simulink model "BajaCVTSim_SimulinkModel"  (R2025a)
settings: Solver=VariableStepAuto  StartTime=0.0  StopTime=30  RelTol=1e-2
model workspace (MAT data in the model file):
  CG = 19.90914
  Cd = 8.5
  Helix = 30
  I_high = 0.9
  I_low = 3.9
  Id_set = 1800
  LR_set = 2400
  L_link = 1.23
  RD_set = 3800
  R_gear = 6.3
  R_helix = 1.455
  R_link = 1.6
  Ramp = 18
  Rfly_max = 1.5
  Rfly_min = 1.89
  Rp_end = 2.775
  Rp_int = 0.975
  Rp_max = 0.975
  Rp_min = 2.775
  Rs_end = 2.4975
  Rs_int = 3.8025
  Rs_max = 2.4975
  Rs_min = 3.8025
  SS_set = 3000
  U = 0.13
  X_0 = 0.975
  X_max = 0.8
  Y_0 = 1.44
  Y_max = 0.8
  axle_F = 32.19442
  axle_R = 29.813464567
  eng_rpm = [1600 1800 2000 2200 2400 2600 2800 3000 3200 3400 3600 4000]
  eng_trq = [15.4 16.5 17.5 18.2 18.5 18.1 17.4 16.6 15.4 14.5 13.5 10]
  kp_lr = 43.75
  ks_lr = 21.25
  ks_tr = 0.592
  m_fly = 120
  m_link = 40
  m_ve = 600
  n_arm = 4
  phi_0 = 100
  phi_max = 40
  theta = 15
  tr = 11
libraries: fl_lib x12, sdl_lib x10, nesl_utility x10, SignalEditorBlockLib x1
settings Model: SimulationMode=accelerator  Creator=jkiss  LastModifiedBy=jkiss
settings DataIOCC: SaveFormat=Array  DSMLogging=off  ReturnWorkspaceOutputs=off

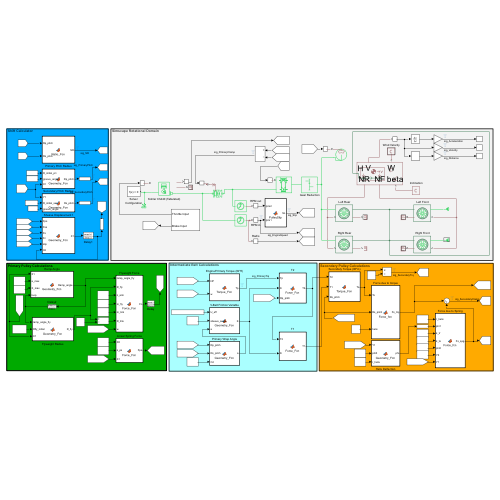
[thumbnail: Simulink's stored preview of the top-level diagram]
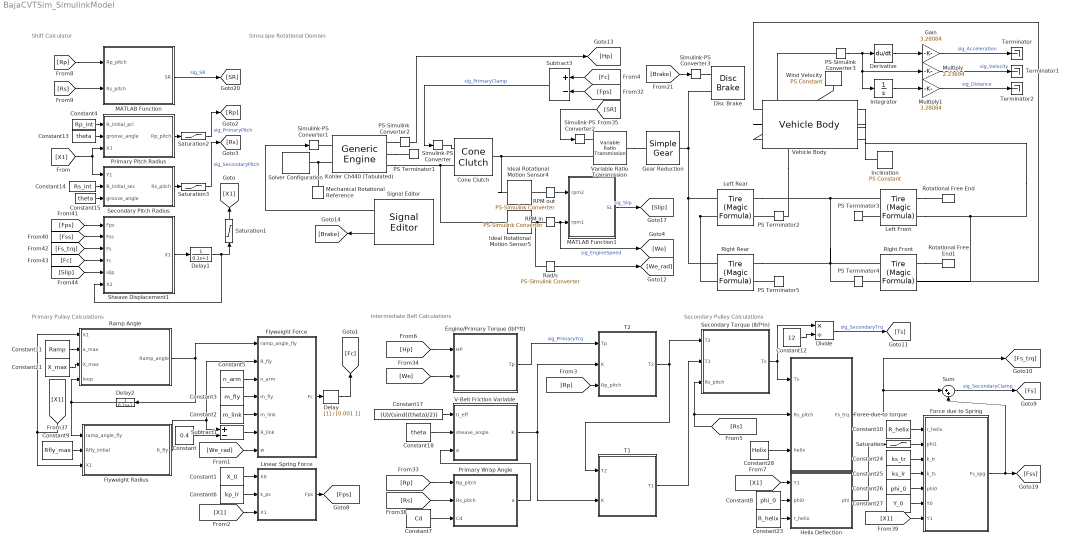
== system BajaCVTSim_SimulinkModel ==
  note: Primary Pulley Calculations
  note: Intermediate Belt Calculations
  note: Secondary Pulley Calculations
  note: Simscape Rotational Domain
  note: Shift Calculator
  Cone Clutch : sdl_lib/Clutches/Cone Clutch  d_o=Rp_end in  d_i=Rp_int in  theta=theta deg  shift_linkage=sdl.enum.shift_linkage.PS  back_stop=true  ring_hub_gap=3 mm  transl_stiffness=10e5 N/m  transl_damping=1e3 N*s/m  visc_fric_transl=100 N*s/m  direction=sdl.enum.shift_linkage_direction.positive  friction_model=sdl.enum.friction_model_TLU_thermal.fixed  mu_w_vector=[0, 100, 1000] rad/s  temperature_TLU=[280, 300, 320] K  mu_static=(U)/(sind((theta)/2))  mu_static_vector=[.4, .38, .36]  mu_coulomb=(U)/(sind((theta)/2))-0.1  mu_coulomb_vector=[.3, .22, .19]  mu_coulomb_temp_vector=[.3, .28, .25]  mu_coulomb_matrix=[.34, .32, .3; .3, .28, .25; .25, .2, .15]  mu_interp_method=simscape.enum.interpolation.linear  mu_extrap_method=simscape.enum.extrapolation.linear  w_tol=0.1 rpm  force_min=X_0*kp_lr lbf  mu_visc=0 N*m*s/rad  initial_state_locked=sdl.enum.initial_lock.unlocked  init_pos=0 mm  thermal_mass=50 kJ/K  T_init=300 K
      settings: InternalSimscapePortConfiguration="{\"Bottom\":[],\"Left\":[{\"id\":\"N\",\"label\":\"N\",\"type\":\"input\"},{\"id\":\"B\",\"label\":\"B\",\"type\":\"foundation.mechanical.rotational.rotational\"}],\"Right\":[{\"id\":\"F\",\"label\":\"F\",\"type\":\"foundation.mechanical.rotational.rotational\"}],\"Top\":[]}"
  Constant : Constant  Value=0.4
  Constant1 : Constant  Value=X_0
  Constant10 : Constant  Value=R_helix
  Constant11 : Constant  Value=Ramp
  Constant12 : Constant  Value=12
  Constant13 : Constant  Value=theta
  Constant14 : Constant  Value=Rs_int
  Constant15 : Constant  Value=theta
  Constant17 : Constant  Value=(U)/(sind((theta)/2))
  Constant18 : Constant  Value=theta
  Constant2 : Constant  Value=m_link
  Constant21 : Constant  Value=X_max
  Constant23 : Constant  Value=R_helix
  Constant24 : Constant  Value=ks_tr
  Constant25 : Constant  Value=ks_lr
  Constant26 : Constant  Value=phi_0
  Constant27 : Constant  Value=Y_0
  Constant28 : Constant  Value=Helix
  Constant3 : Constant  Value=m_fly
  Constant4 : Constant  Value=Rp_int
  Constant5 : Constant  Value=n_arm
  Constant6 : Constant  Value=kp_lr
  Constant7 : Constant  Value=Cd
  Constant8 : Constant  Value=phi_0
  Constant9 : Constant  Value=Rfly_max
  Delay : TransferFcn  Denominator=[0.001 1]
  Delay1 : TransferFcn  Denominator=[0.1 1]
  Delay2 : TransferFcn  Denominator=[0.1 1]
  Derivative : Derivative
  Disc Brake : sdl_lib/Brakes & Detents/Rotational/Disc Brake  r_mean=150 mm  bore=10 mm  n_pads=4  thermal_port=simscape.enum.thermaleffects.omit  mu_static=0.9  mu_coulomb=0.7  temperature_TLU=[280, 300, 320] K  mu_static_TLU=[.9, .8, .7]  mu_coulomb_TLU=[.8, .7, .6]  brkwy_vel=0.1 rpm  visc_coef=0 N*m*s/rad  thermal_mass=50 kJ/K  temperature_specify=off  temperature_priority=High  temperature=300 K  temperature_nominal_specify=off  temperature_nominal_value=1  temperature_nominal_unit=K
  Divide : Product  Inputs=*/
  Engine/Primary Torque (lbf*ft) : MATLAB Function  TreatAsAtomicUnit=on
  Flyweight Force : MATLAB Function  TreatAsAtomicUnit=on
  Flyweight Radius : MATLAB Function  TreatAsAtomicUnit=on
  Force due to Spring : MATLAB Function  TreatAsAtomicUnit=on
  Force due to torque : MATLAB Function  TreatAsAtomicUnit=on
  Gain : Gain  Gain=3.28084
  Gear Reduction : sdl_lib/Gears/Simple Gear  ratio=R_gear  rotation_direction=sdl.enum.shaftOutputDirection.same  friction_model=sdl.enum.gear_efficiencies_load.off  T_noload=0.1 N*m  T_nom=5 N*m  efficiency_nom=0.8  efficiency=0.8  temperature_TLU=[280, 300, 320] K  load_TLU=[1, 5, 10] N*m  efficiency_TLU=[.95, .9, .85]  efficiency_TLU2=[.85, .8, .75; .95, .9, .85; .85, .8, .7]  w_thr=0.01 rad/s  pwr_thr=0.001 W  enable_backlash=false  hardstop_model=simscape.enum.hardstop.smooth  backlash_distance=1e-3 mm  r_base=0.1 m  transition=1e-4 mm  backlash_stiffness=1e6 N/m  backlash_damping=1e3 N*s/m  coeff_rest=0.7  v_tol=0.001 m/s  f_tol=0.001 N  mu_visc=[0, 0] N*m*s/rad  thermal_mass=50 J/K  temperature_specify=off  temperature_priority=High  temperature=300 K  temperature_nominal_specify=off  temperature_nominal_value=1  temperature_nominal_unit=K  x_backlash_specify=off  x_backlash_priority=None  x_backlash=0 mm  x_backlash_nominal_specify=off  x_backlash_nominal_value=1  x_backlash_nominal_unit=mm  f_hardstop_specify=off  f_hardstop_priority=None  f_hardstop=0 N  f_hardstop_nominal_specify=off  f_hardstop_nominal_value=1  f_hardstop_nominal_unit=N  v_backlash_specify=off  v_backlash_priority=None  v_backlash=0 m/s  v_backlash_nominal_specify=off  v_backlash_nominal_value=1  v_backlash_nominal_unit=m/s
  Helix Deflection : MATLAB Function  TreatAsAtomicUnit=on
  Ideal Rotational Motion Sensor4 : fl_lib/Mechanical/Mechanical Sensors/Ideal Rotational Motion Sensor  reference=foundation.enum.MeasurementReference.absolute  acceleration_port=false  velocity_port=true  position_port=false  wrap_angle=false  offset=0 rad
      settings: InternalSimscapePortConfiguration="{\"Bottom\":[],\"Left\":[{\"id\":\"R\",\"label\":\"R\",\"type\":\"foundation.mechanical.rotational.rotational\"}],\"Right\":[{\"id\":\"W\",\"label\":\"W\",\"type\":\"output\"}],\"Top\":[]}"
  Ideal Rotational Motion Sensor5 : fl_lib/Mechanical/Mechanical Sensors/Ideal Rotational Motion Sensor  reference=foundation.enum.MeasurementReference.absolute  acceleration_port=false  velocity_port=true  position_port=false  wrap_angle=false  offset=0 rad
      settings: InternalSimscapePortConfiguration="{\"Bottom\":[],\"Left\":[{\"id\":\"R\",\"label\":\"R\",\"type\":\"foundation.mechanical.rotational.rotational\"}],\"Right\":[{\"id\":\"W\",\"label\":\"W\",\"type\":\"output\"}],\"Top\":[]}"
  Inclination : fl_lib/Physical Signals/Sources/PS Constant  constant=0 rad
  Integrator : Integrator
  Kohler Ch440 (Tabulated) : sdl_lib/Engines & Motors/Generic Engine  input_type=sdl.enum.GenericEngineInputType.NormalizedThrottle  model_parameterization=sdl.enum.engineParameterization.torque  engine_type=sdl.enum.engineType.SI  Trq_max=380 N*m  w_Trq_max=4300 rpm  P_max=9.48 HP_DIN  w_P_max=3000 rpm  w_max=3900 rpm  w_min=0 rpm  w_tab=eng_rpm rpm  trq_tab=eng_trq ft*lb  pwr_tab=[3, 3.2, 3.5, 3.7, 4, 4.7, 5.8, 6.8, 7.6, 8.5, 9, 9.3, 9.5, 9.45, 9.4, 9.3 7] HP_DIN  interp_method=simscape.enum.interpolation.smooth  w_thr=500 rpm  model_inertia=sdl.enum.model_inertia.on  inertia=0.001 kg*m^2  initial_velocity=Id_set rpm  model_time_constant=sdl.enum.lagOffOn.off  time_constant=1 s  initial_normalized_throttle=0  fc_model=sdl.enum.fuel_consumption_model.FuelOff  fc_per_rev=25 mg/rev  fc_w_tab=[1000, 2000, 3000, 4000, 5000, 6000] rpm  fc_trq_tab=[0, 80, 160, 200, 240, 320, 360, 400] N*m  fc_tab=[.5, .9, 1.4, 1.6, 1.9, 2.7, 3.4, 4.4; 1, 1.7, 2.7, 3.1, 3.6, 5, 6, 7.4; 1.4, 2.7, 4, 4.8, 5.6, 7.5, 8.5, 10.5; 2, 3.6, 5.8, 6.7, 8, 10.4, 11.7, 13.3; 2.5, 4.8, 7.9, 9.4, 10.8, 14, 16.2, 18.6; 3.1, 6, 10.3, 11.9, 13.8, 18.4, 22, 26.5] g/s  bmep_tab=[0, 250, 500, 625, 750, 1000, 1150, 1250] kPa  bsfc_tab=[410, 380, 300, 280, 270, 290, 320, 380; 410, 370, 290, 270, 260, 270, 285, 320; 415, 380, 290, 275, 265, 270, 270, 300; 420, 390, 310, 290, 285, 280, 280, 285; 430, 410, 340, 320, 310, 300, 310, 320; 450, 430, 370, 340, 330, 330, 350, 380] g/(hr*kW)  fc_interp_method=simscape.enum.interpolation.linear  displaced_volume=400 cm^3  rev_per_cycle=2  idle_speed=true  idle_speed_reference=Id_set rpm  tau_controller=1 s  idle_w_thr=1 rpm  redline=true  redline_speed=RD_set + 200 rpm  tau_redline=0.01 s  redline_w_thr=10 rpm
      settings: InternalSimscapePortConfiguration="{\"Bottom\":[],\"Left\":[{\"id\":\"ThrNorm\",\"label\":\"Thr\",\"type\":\"input\"},{\"id\":\"B\",\"label\":\"B\",\"type\":\"foundation.mechanical.rotational.rotational\"}],\"Right\":[{\"id\":\"P\",\"label\":\"P\",\"type\":\"output\"},{\"id\":\"FC\",\"label\":\"FC\",\"type\":\"output\"},{\"id\":\"F\",\"label\":\"F\",\"type\":\"foundation.mechanical.rotational.rotational\"}],\"Top\":[]}"
  Left Front : sdl_lib/Tires & Vehicles/Tire (Magic Formula)  parameterization=1  F_z1=2060 N  F_x1=1260 N  kappa1=1  B_m=10  C_m=1.9  D_m=1  E_m=0.97  fz0=2060 N  p_Cx=1.685  p_Dx=[1.21, -.037]  p_Ex=[.344, .095, -.02, 0]  p_Kx=[21.51, -.163, .245]  p_Hx=[-.002, .002]  p_Vx=[0, 0]  rolling_radius_model=sdl.enum.RollingRadiusParameterization.Constant  r_e=tr in  r_0=0.3 m  breff=8.39  dreff=0.26  freff=0.074  q_re0=0.99  q_v1=0.008  longvl=17 m/s  cz=5e5 N/m  model_resistance=false  resistance_model=1  coeff=0.001  p_tire=250e3 Pa  alpha=-0.003  beta=0.97  coeff_a=84e-4  coeff_b=6.2e-4 s/m  coeff_c=1.6e-4 s^2/m^2  p_tire0=240e3 Pa  fz0_resistance=4000 N  vH0=16 m/s  q_Sy=[.0082, 0, .0014, .001, 0, 0, 1.08, -.5]  v_thr=0.1 m/s  enable_scaling_coefficients=false  lfzO=1  lcx=1  lmux=1  lex=1  lkx=1  lhx=1  lvx=1  lmy=1  model_compliance=0  stiffness=1e6 N/m  damping=1000 N/(m/s)  model_inertia=sdl.enum.model_inertia.off  inertia=1e-2 kg*m^2  initial_velocity=0 rpm  vxlow=0.1 m/s  v_tr_thr=0.1*(0.1) m/s  kpumin=-5  kpumax=5
  Left Rear : sdl_lib/Tires & Vehicles/Tire (Magic Formula)  parameterization=sdl.enum.magic_tire_model.peak  F_z1=2060 N  F_x1=1260 N  kappa1=1  B_m=10  C_m=1.9  D_m=1  E_m=0.97  fz0=4000 N  p_Cx=1.685  p_Dx=[1.21, -.037]  p_Ex=[.344, .095, -.02, 0]  p_Kx=[21.51, -.163, .245]  p_Hx=[-.002, .002]  p_Vx=[0, 0]  rolling_radius_model=sdl.enum.RollingRadiusParameterization.Constant  r_e=tr in  r_0=0.3 m  breff=8.39  dreff=0.26  freff=0.074  q_re0=0.99  q_v1=0.008  longvl=17 m/s  cz=5e5 N/m  model_resistance=false  resistance_model=1  coeff=0.001  p_tire=250e3 Pa  alpha=-0.003  beta=0.97  coeff_a=84e-4  coeff_b=6.2e-4 s/m  coeff_c=1.6e-4 s^2/m^2  p_tire0=240e3 Pa  fz0_resistance=4000 N  vH0=16 m/s  q_Sy=[.0082, 0, .0014, .001, 0, 0, 1.08, -.5]  v_thr=0.1 m/s  enable_scaling_coefficients=false  lfzO=1  lcx=1  lmux=1  lex=1  lkx=1  lhx=1  lvx=1  lmy=1  model_compliance=0  stiffness=1e6 N/m  damping=1000 N/(m/s)  model_inertia=sdl.enum.model_inertia.off  inertia=1e-2 kg*m^2  initial_velocity=0 rpm  vxlow=0.1 m/s  v_tr_thr=0.1 m/s  kpumin=-5  kpumax=5
  Linear Spring Force : MATLAB Function  TreatAsAtomicUnit=on
  MATLAB Function : MATLAB Function  TreatAsAtomicUnit=on
  MATLAB Function1 : MATLAB Function  TreatAsAtomicUnit=on
  Mechanical Rotational Reference : fl_lib/Mechanical/Rotational Elements/Mechanical Rotational Reference
  Multiply : Gain  Gain=2.23694
  Multiply1 : Gain  Gain=3.28084
  PS Terminator{1..5} (5 alike) : fl_lib/Physical Signals/Sinks/PS Terminator
  PS-Simulink Converter2 : nesl_utility/PS-Simulink Converter  PhysicalDomain=network_engine_domain  SubClassName=ps_output  LeftPortType=input  RightPortType=output  PseudoPeriodic=off  Frequencies=[]  VectorFormat=inherit  Unit=HP_DIN  AffineConversion=off
  PS-Simulink Converter3 : nesl_utility/PS-Simulink Converter  PhysicalDomain=network_engine_domain  SubClassName=ps_output  LeftPortType=input  RightPortType=output  PseudoPeriodic=off  Frequencies=[]  VectorFormat=1-D array  Unit=m/s  AffineConversion=off
  Primary Pitch Radius : MATLAB Function  TreatAsAtomicUnit=on
  Primary Wrap Angle : MATLAB Function  TreatAsAtomicUnit=on
  RPM in : nesl_utility/PS-Simulink Converter  PhysicalDomain=network_engine_domain  SubClassName=ps_output  LeftPortType=input  RightPortType=output  PseudoPeriodic=off  Frequencies=[]  VectorFormat=inherit  Unit=rpm  AffineConversion=off
  RPM out : nesl_utility/PS-Simulink Converter  PhysicalDomain=network_engine_domain  SubClassName=ps_output  LeftPortType=input  RightPortType=output  PseudoPeriodic=off  Frequencies=[]  VectorFormat=inherit  Unit=rpm  AffineConversion=off
  Rad/s : nesl_utility/PS-Simulink Converter  PhysicalDomain=network_engine_domain  SubClassName=ps_output  LeftPortType=input  RightPortType=output  PseudoPeriodic=off  Frequencies=[]  VectorFormat=inherit  Unit=rad/s  AffineConversion=off
  Ramp Angle : MATLAB Function  TreatAsAtomicUnit=on
  Right Front : sdl_lib/Tires & Vehicles/Tire (Magic Formula)  parameterization=1  F_z1=2060 N  F_x1=1260 N  kappa1=1  B_m=10  C_m=1.9  D_m=1  E_m=0.97  fz0=4000 N  p_Cx=1.685  p_Dx=[1.21, -.037]  p_Ex=[.344, .095, -.02, 0]  p_Kx=[21.51, -.163, .245]  p_Hx=[-.002, .002]  p_Vx=[0, 0]  rolling_radius_model=sdl.enum.RollingRadiusParameterization.Constant  r_e=tr in  r_0=0.3 m  breff=8.39  dreff=0.26  freff=0.074  q_re0=0.99  q_v1=0.008  longvl=17 m/s  cz=5e5 N/m  model_resistance=false  resistance_model=1  coeff=0.001  p_tire=250e3 Pa  alpha=-0.003  beta=0.97  coeff_a=84e-4  coeff_b=6.2e-4 s/m  coeff_c=1.6e-4 s^2/m^2  p_tire0=240e3 Pa  fz0_resistance=4000 N  vH0=16 m/s  q_Sy=[.0082, 0, .0014, .001, 0, 0, 1.08, -.5]  v_thr=0.1 m/s  enable_scaling_coefficients=false  lfzO=1  lcx=1  lmux=1  lex=1  lkx=1  lhx=1  lvx=1  lmy=1  model_compliance=0  stiffness=1e6 N/m  damping=1000 N/(m/s)  model_inertia=sdl.enum.model_inertia.off  inertia=1e-2 kg*m^2  initial_velocity=0 rpm  vxlow=0.1 m/s  v_tr_thr=0.1*(0.1) m/s  kpumin=-5  kpumax=5
  Right Rear : sdl_lib/Tires & Vehicles/Tire (Magic Formula)  parameterization=sdl.enum.magic_tire_model.peak  F_z1=2060 N  F_x1=1260 N  kappa1=1  B_m=10  C_m=1.9  D_m=1  E_m=0.97  fz0=4000 N  p_Cx=1.685  p_Dx=[1.21, -.037]  p_Ex=[.344, .095, -.02, 0]  p_Kx=[21.51, -.163, .245]  p_Hx=[-.002, .002]  p_Vx=[0, 0]  rolling_radius_model=sdl.enum.RollingRadiusParameterization.Constant  r_e=tr in  r_0=0.3 m  breff=8.39  dreff=0.26  freff=0.074  q_re0=0.99  q_v1=0.008  longvl=17 m/s  cz=5e5 N/m  model_resistance=false  resistance_model=1  coeff=0.001  p_tire=250e3 Pa  alpha=-0.003  beta=0.97  coeff_a=84e-4  coeff_b=6.2e-4 s/m  coeff_c=1.6e-4 s^2/m^2  p_tire0=240e3 Pa  fz0_resistance=4000 N  vH0=16 m/s  q_Sy=[.0082, 0, .0014, .001, 0, 0, 1.08, -.5]  v_thr=0.1 m/s  enable_scaling_coefficients=false  lfzO=1  lcx=1  lmux=1  lex=1  lkx=1  lhx=1  lvx=1  lmy=1  model_compliance=0  stiffness=1e6 N/m  damping=1000 N/(m/s)  model_inertia=sdl.enum.model_inertia.off  inertia=1e-2 kg*m^2  initial_velocity=0 rpm  vxlow=0.1 m/s  v_tr_thr=0.1 m/s  kpumin=-5  kpumax=5
  Rotational Free End : fl_lib/Mechanical/Rotational Elements/Rotational Free End  w_specify=off  w_priority=None  w=0 rad/s  w_nominal_specify=off  w_nominal_value=1  w_nominal_unit=rad/s
  Rotational Free End1 : fl_lib/Mechanical/Rotational Elements/Rotational Free End  w_specify=off  w_priority=None  w=0 rad/s  w_nominal_specify=off  w_nominal_value=1  w_nominal_unit=rad/s
  Saturation : Saturate  UpperLimit=phi_0 + phi_max  LowerLimit=phi_0
  Saturation1 : Saturate  UpperLimit=X_max  LowerLimit=0
  Saturation2 : Saturate  UpperLimit=Rp_end  LowerLimit=Rp_int
  Saturation3 : Saturate  UpperLimit=Rs_int  LowerLimit=Rs_end
  Secondary Pitch Radius : MATLAB Function  TreatAsAtomicUnit=on
  Secondary Torque (lbf*in) : MATLAB Function  TreatAsAtomicUnit=on
  Sheave Displacement1 : MATLAB Function  TreatAsAtomicUnit=on
  Signal Editor : SignalEditorBlockLib/Signal Editor  FileName=BajaCVTSim_ThrottleInputs.mat  ActiveScenario=IDLE_50  ActiveSignal=Throttle Input  IsBus=off  OutputBusObjectStr=Bus: BusObject  SampleTime=0  ZeroCross=off  OutputAfterFinalValue=Holding final value  Unit=inherit  PreserveSignalName=on  ApplySigPropsToAllScenarios=on  ApplySigPropsToAllSignals=off  SignalPropertySource=Dialog parameters
  Simulink-PS Converter : nesl_utility/Simulink-PS Converter  PhysicalDomain=network_engine_domain  SubClassName=ps_input  LeftPortType=input  RightPortType=output  PseudoPeriodic=off  Frequencies=[]  NoiseDistribution=none  NoiseParameters=[]  Unit=lbf  AffineConversion=off  FilteringAndDerivatives=provide  SimscapeFilterOrder=1  InputFilterTimeConstant=0.001  UdotUserProvided=0
  Simulink-PS Converter1 : nesl_utility/Simulink-PS Converter  PhysicalDomain=network_engine_domain  SubClassName=ps_input  LeftPortType=input  RightPortType=output  PseudoPeriodic=off  Frequencies=[]  NoiseDistribution=none  NoiseParameters=[]  Unit=1  AffineConversion=off  FilteringAndDerivatives=provide  SimscapeFilterOrder=1  InputFilterTimeConstant=0.001  UdotUserProvided=0
  Simulink-PS Converter2 : nesl_utility/Simulink-PS Converter  PhysicalDomain=network_engine_domain  SubClassName=ps_input  LeftPortType=input  RightPortType=output  PseudoPeriodic=off  Frequencies=[]  NoiseDistribution=none  NoiseParameters=[]  Unit=1  AffineConversion=off  FilteringAndDerivatives=provide  SimscapeFilterOrder=1  InputFilterTimeConstant=0.001  UdotUserProvided=0
  Simulink-PS Converter3 : nesl_utility/Simulink-PS Converter  PhysicalDomain=network_engine_domain  SubClassName=ps_input  LeftPortType=input  RightPortType=output  PseudoPeriodic=off  Frequencies=[]  NoiseDistribution=none  NoiseParameters=[]  Unit=1  AffineConversion=off  FilteringAndDerivatives=provide  SimscapeFilterOrder=1  InputFilterTimeConstant=0.001  UdotUserProvided=0
  Solver Configuration : nesl_utility/Solver Configuration  PhysicalDomain=network_engine_domain  SubClassName=solver  LeftPortType=input  RightPortType=generic  Tones=[]  Harmonics=[]  SimulateNoise=off  Profile=off  UseLocalSampling=off  EnableSwitchedLinearOptims=on  FrequencyDomain=off  UseCCode=off  RelTol=0.001  AbsTol=1e-06  MinStep=1e-09  ToWorkspace=off  RevertToSquareIcSolve=off  NumHomotopyIterations=100  PhasorMode=off  PhasorModeNumHarmonics=1  ConsistencySolver=NEWTON_XTOL_AFTER_FTOL  IndexReductionMethod=DerivativeReplacement  DoDC=off  ResidualTolerance=1e-09  ConsistencyTolSource=GLOBAL  ConsistencyAbsTol=0.001  ConsistencyRelTol=0.001  ConsistencyTolFactor=0.001  UseLocalSolver=off  LocalSolverChoice=NE_BACKWARD_EULER_ADVANCER  ResolveIndetEquations=on  FunctionEvalNumThread=1  LocalSolverSampleTime=0.001  DoFixedCost=off  MaxNonlinIter=3  MaxModeIter=2  ComputeImpulses=off  ImpulseIterations=2  LinearAlgebra=auto  LinearAlgebraNumThread=0  EquationFormulation=NE_TIME_EF  DelaysMemoryBudget=1024  AutomaticFiltering=on  FilteringTimeConstant=0.001  PartitionStorageMethod=AS_NEEDED  PartitionMemoryBudget=1024  PartitionMethod=ROBUST  MultibodyUseLocalSolver=off  MultibodyLocalSolverChoice=ODE1  MultibodyLocalSolverSampleTime=0.001
  Subtract1 : Sum  Inputs=+-
  Subtract3 : Sum  Inputs=+-
  Sum : Sum  Inputs=|++
  T1 : MATLAB Function  TreatAsAtomicUnit=on
  T2 : MATLAB Function  TreatAsAtomicUnit=on
  Terminator : Terminator
  Terminator1 : Terminator
  Terminator2 : Terminator
  V-Belt Friction Variable : MATLAB Function  TreatAsAtomicUnit=on
  Variable Ratio Transmission : sdl_lib/Couplings & Drives/Variable Ratio Transmission  rotation_direction=sdl.enum.shaftOutputDirection.same  kp=1e3 N*m/rad  kv=10 N*m*s/rad  initial_torque=0 N*m  ratio_thr=0.01  losses_model=sdl.enum.lossesOffOn.off  efficiency=0.8  pwr_thr=0.001 W  mu_visc=[0, 0] N*m*s/rad
      settings: InternalSimscapePortConfiguration="{\"Bottom\":[],\"Left\":[{\"id\":\"ratio\",\"label\":\"r\",\"type\":\"input\"},{\"id\":\"B\",\"label\":\"B\",\"type\":\"foundation.mechanical.rotational.rotational\"}],\"Right\":[{\"id\":\"F\",\"label\":\"F\",\"type\":\"foundation.mechanical.rotational.rotational\"}],\"Top\":[]}"
  Vehicle Body : sdl_lib/Tires & Vehicles/Vehicle Body  mass=m_ve lbm  n_w=2  x_f=axle_F in  x_r=axle_R in  y_c=CG+10 in  mass_var=simscape.enum.onoff.off  g=32.2 ft/s^2  liftoff_warning=0  area=.735482 m^2  Cd_var=false  Cd=1.92  rho=1.18 kg/m^3  model_pitch=0  inertia=4000 kg*m^2  suspension_model=1  k_f=1e4 N/m  b_f=1e4 N/(m/s)  k_r=1e4 N/m  b_r=1e4 N/(m/s)  k_f_TLU=[-2000, -1000, 0, 1000, 2000] N  x_f_TLU=[-.4, -.2, 0, .2, .4] m  b_f_TLU=[-200, -100, 0, 100, 200] N  v_f_TLU=[-4, -2, 0, 2, 4] m/s  k_r_TLU=[-2000, -1000, 0, 1000, 2000] N  x_r_TLU=[-.4, -.2, 0, .2, .4] m  b_r_TLU=[-200, -100, 0, 100, 200] N  v_r_TLU=[-4, -2, 0, 2, 4] m/s  interp_method=simscape.enum.interpolation.linear  extrap_method=simscape.enum.extrapolation.linear  model_hardstop=0  upper_bound_f=.25 m  lower_bound_f=-.25 m  stop_k_f=1e6 N/m  stop_b_f=150 N/(m/s)  upper_bound_r=.25 m  lower_bound_r=-.25 m  stop_k_r=1e6 N/m  stop_b_r=150 N/(m/s)  initial_pitch=0 rad  initial_pitch_rate=0 rad/s  v_specify=on  v_priority=High  v=0 m/s  v_nominal_specify=off  v_nominal_value=1  v_nominal_unit=m/s
      settings: InternalSimscapePortConfiguration="{\"Bottom\":[{\"id\":\"NR\",\"label\":\"NR\",\"type\":\"output\"},{\"id\":\"NF\",\"label\":\"NF\",\"type\":\"output\"},{\"id\":\"beta\",\"label\":\"beta\",\"type\":\"input\"}],\"Left\":[{\"id\":\"H\",\"label\":\"H\",\"type\":\"foundation.mechanical.translational.translational\"}],\"Right\":[],\"Top\":[{\"id\":\"V\",\"label\":\"V\",\"type\":\"output\"},{\"id\":\"wind\",\"label\":\"W\",\"type\":\"input\"}]}"
  Wind Velocity : fl_lib/Physical Signals/Sources/PS Constant  constant=0
  wires:
  Signal Editor/2 -> [Brake]
  [Fc] -> Subtract3/1
  MATLAB Function1/1(SL) -> [Slip]  "sig_Slip"
  RPM out/1 -> MATLAB Function1/1(rpm2)
  RPM in/1 -> [We], MATLAB Function1/2(rpm1)  "sig_EngineSpeed"
  Constant5/1 -> Flyweight Force/3(n_arm)
  Constant3/1 -> Flyweight Force/4(m_fly)
  Constant2/1 -> Flyweight Force/5(m_link)
  Flyweight Radius/1(R_fly) -> Subtract1/1, Flyweight Force/2(R_fly)
  Subtract1/1 -> Flyweight Force/6(R_link)
  Constant/1 -> Subtract1/2
  Constant9/1 -> Flyweight Radius/2(Rfly_initial)
  [X1] -> Ramp Angle/1(X1), Flyweight Radius/3(X1)
  Ramp Angle/1(Ramp_angle) -> Flyweight Force/1(ramp_angle_fly), Delay2/1
  Constant11/1 -> Ramp Angle/2(a_max)
  Constant21/1 -> Ramp Angle/3(X_max)
  [X1] -> Linear Spring Force/3(X1)
  Constant1/1 -> Linear Spring Force/1(X0)
  Constant6/1 -> Linear Spring Force/2(k_ps)
  Flyweight Force/1(Fc) -> Delay/1
  Rad/s/1 -> [We_rad]
  T2/1(T2) -> T1/1(T2), Secondary Torque (lbf*in)/1(T2)
  Delay/1 -> [Fc]
  T1/1(T1) -> Secondary Torque (lbf*in)/2(T1)
  Linear Spring Force/1(Fps) -> [Fps]
  [Rs] -> Primary Wrap Angle/2(Rs_pitch)
  [Rp] -> Primary Wrap Angle/1(Rp_pitch)
  [Rs] -> Secondary Torque (lbf*in)/3(Rs_pitch), Force due to torque/2(Rs_pitch)
  [Rp] -> T2/3(Rp_pitch)
  Constant10/1 -> Force due to Spring/1(r_helix)
  Constant8/1 -> Helix Deflection/2(phi0)
  Constant23/1 -> Helix Deflection/3(r_helix)
  Helix Deflection/1(phi) -> Saturation/1
  Constant18/1 -> V-Belt Friction Variable/2(sheave_angle)
  Constant26/1 -> Force due to Spring/5(phi0)
  Constant24/1 -> Force due to Spring/3(k_tr)
  Constant25/1 -> Force due to Spring/4(k_ts)
  Constant27/1 -> Force due to Spring/6(Y0)
  Constant7/1 -> Primary Wrap Angle/3(Cd)
  Signal Editor/1 -> Simulink-PS Converter1/1
  [Fps] -> Subtract3/2
  Subtract3/1 -> Simulink-PS Converter/1  "sig_PrimaryClamp"
  [We] -> Engine/Primary Torque (lbf*ft)/2(w)
  PS-Simulink Converter2/1 -> [Hp]
  [Hp] -> Engine/Primary Torque (lbf*ft)/1(HP)
  [SR] -> Simulink-PS Converter2/1
  PS-Simulink Converter3/1 -> Derivative/1, Integrator/1, Multiply/1
  Multiply/1 -> Terminator1/1  "sig_Velocity"
  Integrator/1 -> Multiply1/1
  Multiply1/1 -> Terminator2/1  "sig_Distance"
  [Brake] -> Simulink-PS Converter3/1
  [We_rad] -> Flyweight Force/7(w)
  Primary Wrap Angle/1(a) -> V-Belt Friction Variable/3(a)
  Constant17/1 -> V-Belt Friction Variable/1(U_eff)
  V-Belt Friction Variable/1(K) -> T1/2(K), T2/2(K)
  Engine/Primary Torque (lbf*ft)/1(Tp) -> T2/1(Tp)  "sig_PrimaryTrq"
  Divide/1 -> [Ts]  "sig_SecondaryTrq"
  [X1] -> Helix Deflection/1(Y1)
  Saturation/1 -> Force due to Spring/2(phi1)
  Force due to torque/1(Fs_trq) -> [Fs_trq], Sum/1
  Sum/1 -> [Fs]  "sig_SecondaryClamp"
  Force due to Spring/1(Fs_spg) -> [Fss], Sum/2
  [X1] -> Force due to Spring/7(Y1)
  [Fss] -> Sheave Displacement1/2(Fss)
  [Fs_trq] -> Sheave Displacement1/3(Fs)
  [Fps] -> Sheave Displacement1/1(Fps)
  [Fc] -> Sheave Displacement1/4(Fc)
  [Slip] -> Sheave Displacement1/5(slip)
  Delay1/1 -> Sheave Displacement1/6(X2), Saturation1/1
  Sheave Displacement1/1(X1) -> Delay1/1
  Constant13/1 -> Primary Pitch Radius/2(groove_angle)
  Primary Pitch Radius/1(Rp_pitch) -> Saturation2/1
  Constant4/1 -> Primary Pitch Radius/1(R_initial_pri)
  Constant14/1 -> Secondary Pitch Radius/2(R_initial_sec)
  Constant15/1 -> Secondary Pitch Radius/3(groove_angle)
  Secondary Pitch Radius/1(Rs_pitch) -> Saturation3/1
  MATLAB Function/1(SR) -> [SR]  "sig_SR"
  Constant28/1 -> Force due to torque/3(helix)
  Delay2/1 -> Ramp Angle/4(loop), Flyweight Radius/1(ramp_angle_fly)
  Secondary Torque (lbf*in)/1(Ts) -> Divide/1, Force due to torque/1(Ts)
  Constant12/1 -> Divide/2
  Derivative/1 -> Gain/1
  Gain/1 -> Terminator/1  "sig_Acceleration"
  Saturation2/1 -> [Rp]  "sig_PrimaryPitch"
  Saturation3/1 -> [Rs]  "sig_SecondaryPitch"
  [X1] -> Primary Pitch Radius/3(X1), Secondary Pitch Radius/1(Y1)
  [Rs] -> MATLAB Function/2(Rs_pitch)
  [Rp] -> MATLAB Function/1(Rp_pitch)
  Saturation1/1 -> [X1]
  connections:
  Kohler Ch440 (Tabulated)/LConn2 -- Solver Configuration/RConn1 -- Mechanical Rotational Reference/LConn1
  Ideal Rotational Motion Sensor5/LConn1 -- Kohler Ch440 (Tabulated)/RConn3 -- Cone Clutch/LConn2
  Rad/s/LConn1 -- Ideal Rotational Motion Sensor5/RConn1 -- RPM in/LConn1
  Ideal Rotational Motion Sensor4/LConn1 -- Cone Clutch/RConn1 -- Variable Ratio Transmission/LConn2
  Simulink-PS Converter/RConn1 -- Cone Clutch/LConn1
  RPM out/LConn1 -- Ideal Rotational Motion Sensor4/RConn1
  Right Rear/LConn2 -- Left Rear/LConn2 -- Gear Reduction/RConn1 -- Disc Brake/LConn2
  Simulink-PS Converter2/RConn1 -- Variable Ratio Transmission/LConn1
  Variable Ratio Transmission/RConn1 -- Gear Reduction/LConn1
  Kohler Ch440 (Tabulated)/LConn1 -- Simulink-PS Converter1/RConn1
  Kohler Ch440 (Tabulated)/RConn1 -- PS-Simulink Converter2/LConn1
  Kohler Ch440 (Tabulated)/RConn2 -- PS Terminator1/LConn1
  Left Rear/LConn1 -- Vehicle Body/RConn1 -- Right Rear/LConn1
  Right Front/RConn2 -- Vehicle Body/LConn1 -- Right Rear/RConn2 -- Left Rear/RConn2 -- Left Front/RConn2
  Left Front/LConn1 -- Vehicle Body/RConn2 -- Right Front/LConn1
  Vehicle Body/RConn3 -- Inclination/RConn1
  Left Front/RConn1 -- PS Terminator3/LConn1
  Simulink-PS Converter3/RConn1 -- Disc Brake/LConn1
  Left Front/LConn2 -- Rotational Free End/LConn1
  Right Front/RConn1 -- PS Terminator4/LConn1
  Vehicle Body/LConn3 -- Wind Velocity/RConn1
  Right Front/LConn2 -- Rotational Free End1/LConn1
  Vehicle Body/LConn2 -- PS-Simulink Converter3/LConn1
  PS Terminator2/LConn1 -- Left Rear/RConn1
  PS Terminator5/LConn1 -- Right Rear/RConn1

== matlab function BajaCVTSim_SimulinkModel/Linear Spring Force ==
  data: X0 input; k_ps input; X1 input; Fps output
function Fps = Force_Fcn(X0,k_ps,X1)

Fps = k_ps*(X0 + X1);

end

== matlab function BajaCVTSim_SimulinkModel/Secondary Torque (lbf*in) ==
  data: T2 input; Ts output; T1 input; Rs_pitch input
function Ts = Torque_Fcn(T2,T1,Rs_pitch)

Ts = (T1-T2)*Rs_pitch; %lbf*in

end

== matlab function BajaCVTSim_SimulinkModel/Force due to torque ==
  data: Ts input; Rs_pitch input; helix input; Fs_trq output
function Fs_trq = Force_fcn(Ts,Rs_pitch,helix)

Fs_trq = (Ts/Rs_pitch)*tand(helix);

end

== matlab function BajaCVTSim_SimulinkModel/Force due to Spring ==
  data: r_helix input; phi1 input; k_tr input; k_ts input; Fs_spg output; phi0 input; Y0 input; Y1 input
function Fs_spg = Force_fcn(r_helix,phi1,k_tr,k_ts,phi0,Y0,Y1)

Fs_spg = (k_tr*(phi0 + phi1))/(2*r_helix) + (k_ts*(Y0 + Y1));

end

== matlab function BajaCVTSim_SimulinkModel/Flyweight Force ==
  data: ramp_angle_fly input; R_fly input; n_arm input; m_fly input; m_link input; R_link input; w input; Fc output
function Fc = Force_Fcn(ramp_angle_fly,R_fly,n_arm,m_fly,m_link,R_link,w)

Fc = (((m_fly/14593.89567)*n_arm*(R_fly/12) + (m_link/14593.89567)*n_arm*(R_link/12))*(w^2))*tand(ramp_angle_fly);

end

== matlab function BajaCVTSim_SimulinkModel/Sheave Displacement1 ==
  data: Fps input; Fss input; Fs input; Fc input; slip input; X1 output; X2 input
function X1 = Geometry_Fcn(Fps,Fss,Fs,Fc,slip,X2)
    if slip <= 5
        if X2 >= 0.2
            if Fc-Fps > Fs + Fss
                X1 = X2 + 0.0799;
            else
                X1 = X2;
            end
        elseif X2 >= 0.35
            if Fc-Fps > Fs + Fss
                X1 = X2 + 0.01;
            else
                X1 = X2;
            end
        else
            if Fc-Fps > Fs + Fss
                X1 = X2 + 0.08;
            else
                X1 = X2;
            end
        end
    else
        X1 = 0;
    end
end

== matlab function BajaCVTSim_SimulinkModel/Primary Pitch Radius ==
  data: R_initial_pri input; groove_angle input; X1 input; Rp_pitch output
function Rp_pitch = Geometry_Fcn(R_initial_pri,groove_angle,X1)

Rp_pitch = R_initial_pri + (X1)/tand(groove_angle);

end

== matlab function BajaCVTSim_SimulinkModel/Secondary Pitch Radius ==
  data: Y1 input; R_initial_sec input; Rs_pitch output; groove_angle input
function Rs_pitch = Geometry_Fcn(Y1,R_initial_sec,groove_angle)

Rs_pitch = R_initial_sec - (Y1)/tand(groove_angle);

end

== matlab function BajaCVTSim_SimulinkModel/MATLAB Function ==
  data: Rp_pitch input; SR output; Rs_pitch input
function SR = Ratio_Fcn(Rp_pitch,Rs_pitch)

SR = Rs_pitch/Rp_pitch;

end

== matlab function BajaCVTSim_SimulinkModel/Helix Deflection ==
  data: Y1 input; phi0 input; r_helix input; phi output
function phi = Geometry_Fcn(Y1,phi0,r_helix)

phi = 2*(90 - acosd(Y1/r_helix)) + phi0;

end

== matlab function BajaCVTSim_SimulinkModel/Primary Wrap Angle ==
  data: Rp_pitch input; a output; Rs_pitch input; Cd input
function a = Geometry_Fcn(Rp_pitch,Rs_pitch,Cd)

a = pi + 2*asin((Rs_pitch-Rp_pitch)/Cd);

end

== matlab function BajaCVTSim_SimulinkModel/V-Belt Friction Variable ==
  data: U_eff input; sheave_angle input; a input; K output
function K = Geometry_Fcn(U_eff,sheave_angle,a)

K = exp((U_eff*a)/sind(sheave_angle));

end

== matlab function BajaCVTSim_SimulinkModel/T1 ==
  data: T2 input; T1 output; K input
function T1 = Force_Fcn(T2,K)

T1 = T2*K;

end

== matlab function BajaCVTSim_SimulinkModel/MATLAB Function1 ==
  data: rpm2 input; rpm1 input; SL output
function SL = PulleySlip(rpm2,rpm1)

SL = ((rpm1-rpm2)/rpm1) * 100;

end

== matlab function BajaCVTSim_SimulinkModel/T2 ==
  data: Tp input; T2 output; K input; Rp_pitch input
function T2 = Force_Fcn(Tp,K,Rp_pitch)

T2 = (Tp*12)/(Rp_pitch*(K-1));

end

== matlab function BajaCVTSim_SimulinkModel/Ramp Angle ==
  data: X1 input; a_max input; X_max input; Ramp_angle output; loop input
function Ramp_angle = Geometry_Fcn(X1,a_max,X_max,loop)
if X1 >= X_max*0.25
    Ramp_angle = a_max - exp(-4*(0.2-X1)) + 1;
else
    Ramp_angle = a_max;
end
end

== matlab function BajaCVTSim_SimulinkModel/Flyweight Radius ==
  data: ramp_angle_fly input; Rfly_initial input; R_fly output; X1 input
function R_fly = Geometry_Fcn(ramp_angle_fly,Rfly_initial,X1)

R_fly = X1*tand(ramp_angle_fly) + Rfly_initial;

end

== matlab function BajaCVTSim_SimulinkModel/Engine//Primary Torque (lbf*ft) ==
  data: HP input; Tp output; w input
function Tp = Torque_Fcn(HP,w)

Tp = (HP*5252)/w; %lbf*ft

end
